simulink library "motohawk_control_primitives_lib"  (Simulink 7.5)
settings: Solver=ode45  SolverMode=SingleTasking  StartTime=0.0  StopTime=10.0  RelTol=1e-3
undefined symbols (not defined in the file): group, motohawk_vardec_config_group, motohawk_vardec_path, p, samp_time, SampleTime
libraries: MotoHawk_lib x103, motohawk_control_primitives_lib x29, simulink x11, AutoDoc_lib x4
(part 4 of 4)

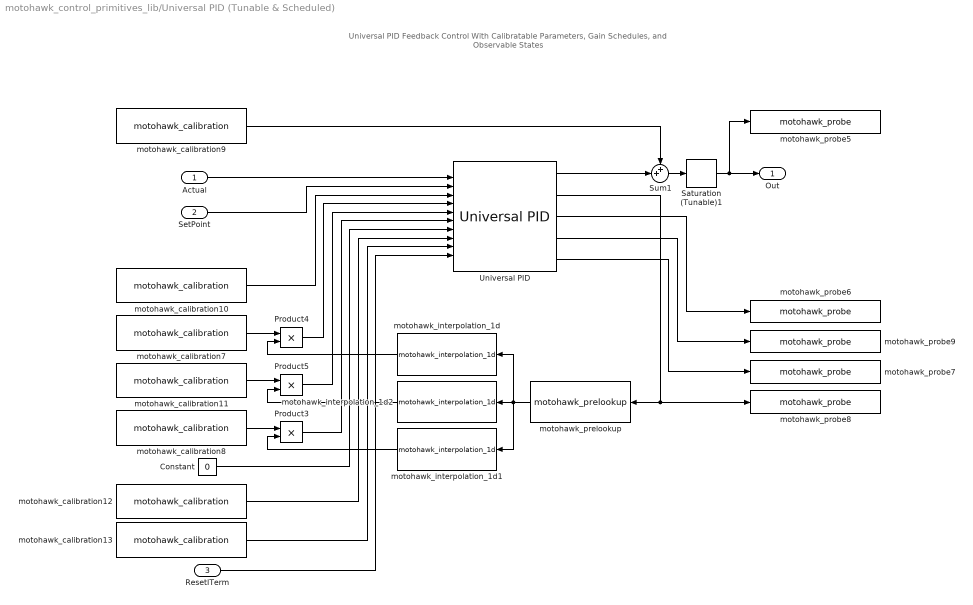
== system motohawk_control_primitives_lib/Universal PID (Tunable & Scheduled) ==
  note: Universal PID Feedback Control
      | With Calibratable Parameters,
      | Gain Schedules, and Observable States
  Actual : Inport  OutDataType=sfix(16)  OutScaling=2^0
  SetPoint : Inport  Port=2  OutDataType=sfix(16)  OutScaling=2^0
  ResetITerm : Inport  Port=3  OutDataType=sfix(16)  OutScaling=2^0
  Constant : Constant  Value=0  OutDataType=sfix(16)  OutScaling=2^0  OutDataTypeStr=Inherit: Inherit via back propagation
  Product3 : Product  OutDataType=sfix(16)  OutScaling=2^0  SaturateOnIntegerOverflow=on  InputSameDT=on  OutDataTypeStr=Inherit: Same as first input
  Product4 : Product  OutDataType=sfix(16)  OutScaling=2^0  SaturateOnIntegerOverflow=on  InputSameDT=on  OutDataTypeStr=Inherit: Same as first input
  Product5 : Product  OutDataType=sfix(16)  OutScaling=2^0  SaturateOnIntegerOverflow=on  InputSameDT=on  OutDataTypeStr=Inherit: Same as first input
  Saturation (Tunable)1 : motohawk_control_primitives_lib/Saturation (Tunable)  prefix=prefix  units=units  grp=motohawk_vardec_config_group(grp)
  Sum1 : Sum  Inputs=++|  OutDataType=sfix(16)  OutScaling=2^0  InputSameDT=on
  Universal PID : motohawk_control_primitives_lib/Universal PID  Description=|  samp_time=SampleTime
      | /* Name: ErrorGain Unit:mult ClassID:VAR StorageID:FLASH Access:RW4+RW3+NA2+NA1 TypeID:UINT4                   
      |    Gain:0.000000001 Min:0.000000000 Max:4.000000000 Format:10.9 UpdateID:REMOTE Help:"This gain is applied to "
      |    "the error term before it is used to calculate the P, I and D terms." VardecSig:6C */                       
      |                                                                                                                
      | /* Name: ITermLowerLim Unit:0 ClassID:VAR StorageID:FLASH Access:RW4+RW3+NA2+NA1 TypeID:SINT2 Gain:0.1         
      |    Min:-3276.8 Max:3276.7 Format:5.1 UpdateID:REMOTE Help:"Lower limit on the I-term value." VardecSig:6C */   
      |                                                                                                                
      | /* Name: ITermUpperLim ClassID:VAR StorageID:FLASH Access:RW4+RW3+NA2+NA1 TypeID:SINT2 Gain:0.1 Min:-3276.8    
      |    Max:3276.7 Format:5.1 UpdateID:REMOTE Help:"Upper limit on I-term value." VardecSig:6C */                   
      |                                                                                                                
      | /* Name: PIDOutLowerLim ClassID:VAR StorageID:FLASH Access:RW4+RW3+NA2+NA1 TypeID:SINT2 Gain:0.1               
      |    Min:-3276.8 Max:3276.7 Format:5.1 UpdateID:REMOTE Help:"Lower limit on PID output." VardecSig:6C */         
      |                                                                                                                
      | /* Name: PIDOutUpperLim ClassID:VAR StorageID:FLASH Access:RW4+RW3+NA2+NA1 TypeID:SINT2 Gain:0.1               
      |    Min:-3276.8 Max:3276.7 Format:3.1 UpdateID:REMOTE Help:"Upper limit on PID output." VardecSig:6C */
  motohawk_calibration10 : MotoHawk_lib/Calibration & Probing Blocks/motohawk_calibration  nam=[prefix 'ErrorGain']  val=1  storage=Calibration  show_more=on  name_source=Use Parameter  data_type=Inherit from 'Default Value'  read_level=1  write_level=1  ovr_cals=on  view_as=Number  enum_struct={'Disabled', 'Enabled'}  vector_style=Wide Row  use_help_units=on  help='PID Error Gain'  units='mult'  use_header_enum=off  row_header_enum={}  col_header_enum={}  use_min_max=off  min_val=-inf  max_val=inf  use_precision=off  precision=''  gain=1  offset=0  exp=1  use_mototune_group=on  mototune_group=motohawk_vardec_config_group(grp)
  motohawk_calibration11 : MotoHawk_lib/Calibration & Probing Blocks/motohawk_calibration  nam=[prefix 'IGain']  val=1  storage=Calibration  show_more=on  name_source=Use Parameter  data_type=Inherit from 'Default Value'  read_level=1  write_level=1  ovr_cals=on  view_as=Number  enum_struct={'Disabled', 'Enabled'}  vector_style=Wide Row  use_help_units=on  help='PID Integrator Gain'  units='mult'  use_header_enum=off  row_header_enum={}  col_header_enum={}  use_min_max=off  min_val=-inf  max_val=inf  use_precision=off  precision=''  gain=1  offset=0  exp=1  use_mototune_group=on  mototune_group=motohawk_vardec_config_group(grp)
  motohawk_calibration12 : MotoHawk_lib/Calibration & Probing Blocks/motohawk_calibration  nam=[prefix 'IMin']  val=0  storage=Calibration  show_more=on  name_source=Use Parameter  data_type=Inherit from 'Default Value'  read_level=1  write_level=1  ovr_cals=on  view_as=Number  enum_struct={'Disabled', 'Enabled'}  vector_style=Wide Row  use_help_units=on  help='PID Integrator Lower Limit'  units=units  use_header_enum=off  row_header_enum={}  col_header_enum={}  use_min_max=off  min_val=-inf  max_val=inf  use_precision=off  precision=''  gain=1  offset=0  exp=1  use_mototune_group=on  mototune_group=motohawk_vardec_config_group(grp)
  motohawk_calibration13 : MotoHawk_lib/Calibration & Probing Blocks/motohawk_calibration  nam=[prefix 'IMax']  val=1  storage=Calibration  show_more=on  name_source=Use Parameter  data_type=Inherit from 'Default Value'  read_level=1  write_level=1  ovr_cals=on  view_as=Number  enum_struct={'Disabled', 'Enabled'}  vector_style=Wide Row  use_help_units=on  help='PID Integrator Upper Limit'  units=units  use_header_enum=off  row_header_enum={}  col_header_enum={}  use_min_max=off  min_val=-inf  max_val=inf  use_precision=off  precision=''  gain=1  offset=0  exp=1  use_mototune_group=on  mototune_group=motohawk_vardec_config_group(grp)
  motohawk_calibration7 : MotoHawk_lib/Calibration & Probing Blocks/motohawk_calibration  nam=[prefix 'PGain']  val=1  storage=Calibration  show_more=on  name_source=Use Parameter  data_type=Inherit from 'Default Value'  read_level=1  write_level=1  ovr_cals=on  view_as=Number  enum_struct={'Disabled', 'Enabled'}  vector_style=Wide Row  use_help_units=on  help='PID Proportional Gain'  units='mult'  use_header_enum=off  row_header_enum={}  col_header_enum={}  use_min_max=off  min_val=-inf  max_val=inf  use_precision=off  precision=''  gain=1  offset=0  exp=1  use_mototune_group=on  mototune_group=motohawk_vardec_config_group(grp)
  motohawk_calibration8 : MotoHawk_lib/Calibration & Probing Blocks/motohawk_calibration  nam=[prefix 'DGain']  val=1  storage=Calibration  show_more=on  name_source=Use Parameter  data_type=Inherit from 'Default Value'  read_level=1  write_level=1  ovr_cals=on  view_as=Number  enum_struct={'Disabled', 'Enabled'}  vector_style=Wide Row  use_help_units=on  help='PID Derivative Gain'  units='mult'  use_header_enum=off  row_header_enum={}  col_header_enum={}  use_min_max=off  min_val=-inf  max_val=inf  use_precision=off  precision=''  gain=1  offset=0  exp=1  use_mototune_group=on  mototune_group=motohawk_vardec_config_group(grp)
  motohawk_calibration9 : MotoHawk_lib/Calibration & Probing Blocks/motohawk_calibration  nam=[prefix 'DCOffset']  val=0  storage=Calibration  show_more=on  name_source=Use Parameter  data_type=Inherit from 'Default Value'  read_level=1  write_level=1  ovr_cals=on  view_as=Number  enum_struct={'Disabled', 'Enabled'}  vector_style=Wide Row  use_help_units=on  help='PID Output DC Offset'  units=units  use_header_enum=off  row_header_enum={}  col_header_enum={}  use_min_max=off  min_val=-inf  max_val=inf  use_precision=off  precision=''  gain=1  offset=0  exp=1  use_mototune_group=on  mototune_group=motohawk_vardec_config_group(grp)
  motohawk_interpolation_1d : MotoHawk_lib/Lookup Tables/motohawk_interpolation_1d  nam=[prefix 'PMult']  table_data=ones(1,tblsize)  show_more=on  data_type=Inherit from 'Table Data'  storage=NonAdaptive  read_level=1  write_level=1  ovr_cals=on  use_help=on  help='Proportional term gain schedule'  units='mult'  use_min_max=off  min_val=-inf  max_val=inf  use_precision=off  precision=''  gain=1  offset=0  exp=1  use_links=off  prelookup_block=''  output_name=''  use_mototune_group=on  mototune_group=grp
  motohawk_interpolation_1d1 : MotoHawk_lib/Lookup Tables/motohawk_interpolation_1d  nam=[prefix 'DMult']  table_data=ones(1,tblsize)  show_more=on  data_type=Inherit from 'Table Data'  storage=NonAdaptive  read_level=1  write_level=1  ovr_cals=on  use_help=on  help='Derivative term gain schedule'  units='mult'  use_min_max=off  min_val=-inf  max_val=inf  use_precision=off  precision=''  gain=1  offset=0  exp=1  use_links=off  prelookup_block=''  output_name=''  use_mototune_group=on  mototune_group=grp
  motohawk_interpolation_1d2 : MotoHawk_lib/Lookup Tables/motohawk_interpolation_1d  nam=[prefix 'IMult']  table_data=ones(1,tblsize)  show_more=on  data_type=Inherit from 'Table Data'  storage=NonAdaptive  read_level=1  write_level=1  ovr_cals=on  use_help=on  help='Integrator term gain schedule'  units='mult'  use_min_max=off  min_val=-inf  max_val=inf  use_precision=off  precision=''  gain=1  offset=0  exp=1  use_links=off  prelookup_block=''  output_name=''  use_mototune_group=on  mototune_group=grp
  motohawk_prelookup : MotoHawk_lib/Lookup Tables/motohawk_prelookup  nam=[prefix 'Error']  breakpoint_data=ones(1,tblsize)  show_more=on  data_type=Inherit from 'Table Data'  storage=Constant  read_level=1  write_level=1  ovr_cals=on  use_help=on  help='Error gain schedule ordinates'  units=units  use_min_max=off  min_val=-inf  max_val=inf  use_precision=off  precision=''  gain=1  offset=0  exp=1  use_links=on  input_name=[prefix 'Error']  use_mototune_group=on  mototune_group=grp
  motohawk_probe5 : MotoHawk_lib/Calibration & Probing Blocks/motohawk_probe  nam=[prefix 'Out']  show_more=on  name_source=Use Parameter  read_level=1  view_as=Number  enum_struct={'Disabled', 'Enabled'}  vector_style=Wide Row  use_help_units=on  help='PID Final Output'  units=units  use_header_enum=off  row_header_enum={}  col_header_enum={}  use_precision=off  precision=''  gain=1  offset=0  exp=1  use_mototune_group=on  mototune_group=grp
  motohawk_probe6 : MotoHawk_lib/Calibration & Probing Blocks/motohawk_probe  nam=[prefix 'PTerm']  show_more=on  name_source=Use Parameter  read_level=1  view_as=Number  enum_struct={'Disabled', 'Enabled'}  vector_style=Wide Row  use_help_units=on  help='PID Proportional Term'  units=units  use_header_enum=off  row_header_enum={}  col_header_enum={}  use_precision=off  precision=''  gain=1  offset=0  exp=1  use_mototune_group=on  mototune_group=grp
  motohawk_probe7 : MotoHawk_lib/Calibration & Probing Blocks/motohawk_probe  nam=[prefix 'DTerm']  show_more=on  name_source=Use Parameter  read_level=1  view_as=Number  enum_struct={'Disabled', 'Enabled'}  vector_style=Wide Row  use_help_units=on  help='PID Derivative Term'  units=units  use_header_enum=off  row_header_enum={}  col_header_enum={}  use_precision=off  precision=''  gain=1  offset=0  exp=1  use_mototune_group=on  mototune_group=grp
  motohawk_probe8 : MotoHawk_lib/Calibration & Probing Blocks/motohawk_probe  nam=[prefix 'Error']  show_more=on  name_source=Use Parameter  read_level=1  view_as=Number  enum_struct={'Disabled', 'Enabled'}  vector_style=Wide Row  use_help_units=on  help='PID Error Term'  units=units  use_header_enum=off  row_header_enum={}  col_header_enum={}  use_precision=off  precision=''  gain=1  offset=0  exp=1  use_mototune_group=on  mototune_group=grp
  motohawk_probe9 : MotoHawk_lib/Calibration & Probing Blocks/motohawk_probe  nam=[prefix 'ITerm']  show_more=on  name_source=Use Parameter  read_level=1  view_as=Number  enum_struct={'Disabled', 'Enabled'}  vector_style=Wide Row  use_help_units=on  help='PID Integrator Term'  units=units  use_header_enum=off  row_header_enum={}  col_header_enum={}  use_precision=off  precision=''  gain=1  offset=0  exp=1  use_mototune_group=on  mototune_group=grp
  Out : Outport  OutDataType=sfix(16)  OutScaling=2^0
  wires:
  motohawk_calibration13/1 -> Universal PID/9
  motohawk_calibration12/1 -> Universal PID/8
  Constant/1 -> Universal PID/7
  ResetITerm/1 -> Universal PID/10
  Universal PID/4 -> motohawk_probe9/1
  Universal PID/3 -> motohawk_probe6/1
  Universal PID/2 -> motohawk_probe8/1, motohawk_prelookup/1
  Product5/1 -> Universal PID/5
  motohawk_interpolation_1d2/1 -> Product5/2
  motohawk_calibration11/1 -> Product5/1
  motohawk_prelookup/1 -> motohawk_interpolation_1d2/1, motohawk_interpolation_1d1/1, motohawk_interpolation_1d/1
  SetPoint/1 -> Universal PID/2
  Actual/1 -> Universal PID/1
  Saturation (Tunable)1/1 -> motohawk_probe5/1, Out/1
  Universal PID/5 -> motohawk_probe7/1
  Universal PID/1 -> Sum1/2
  Sum1/1 -> Saturation (Tunable)1/1
  motohawk_calibration9/1 -> Sum1/1
  motohawk_calibration10/1 -> Universal PID/3
  Product4/1 -> Universal PID/4
  motohawk_calibration7/1 -> Product4/1
  Product3/1 -> Universal PID/6
  motohawk_calibration8/1 -> Product3/1
  motohawk_interpolation_1d/1 -> Product4/2
  motohawk_interpolation_1d1/1 -> Product3/2

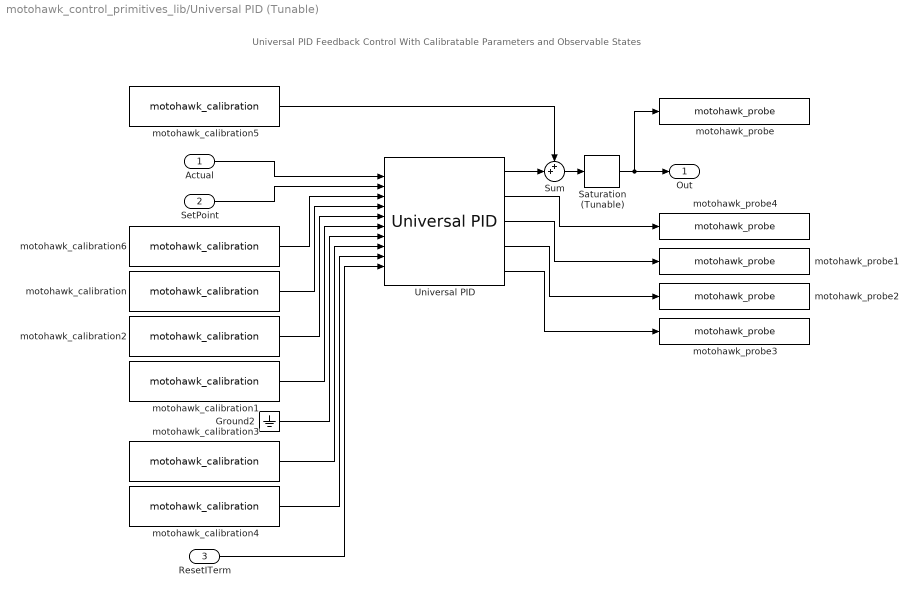
== system motohawk_control_primitives_lib/Universal PID (Tunable) ==
  note: Universal PID Feedback Control
      | With Calibratable Parameters and Observable States
  Actual : Inport  OutDataType=sfix(16)  OutScaling=2^0
  SetPoint : Inport  Port=2  OutDataType=sfix(16)  OutScaling=2^0
  ResetITerm : Inport  Port=3  OutDataType=sfix(16)  OutScaling=2^0
  Ground2 : Ground
  Saturation (Tunable) : motohawk_control_primitives_lib/Saturation (Tunable)  prefix=prefix  units=units  grp=grp
  Sum : Sum  Inputs=++|  OutDataType=sfix(16)  OutScaling=2^0  InputSameDT=on
  Universal PID : motohawk_control_primitives_lib/Universal PID  Description=|  samp_time=SampleTime
      | /* Name: ErrorGain Unit:mult ClassID:VAR StorageID:FLASH Access:RW4+RW3+NA2+NA1 TypeID:UINT4                   
      |    Gain:0.000000001 Min:0.000000000 Max:4.000000000 Format:10.9 UpdateID:REMOTE Help:"This gain is applied to "
      |    "the error term before it is used to calculate the P, I and D terms." VardecSig:6C */                       
      |                                                                                                                
      | /* Name: ITermLowerLim Unit:0 ClassID:VAR StorageID:FLASH Access:RW4+RW3+NA2+NA1 TypeID:SINT2 Gain:0.1         
      |    Min:-3276.8 Max:3276.7 Format:5.1 UpdateID:REMOTE Help:"Lower limit on the I-term value." VardecSig:6C */   
      |                                                                                                                
      | /* Name: ITermUpperLim ClassID:VAR StorageID:FLASH Access:RW4+RW3+NA2+NA1 TypeID:SINT2 Gain:0.1 Min:-3276.8    
      |    Max:3276.7 Format:5.1 UpdateID:REMOTE Help:"Upper limit on I-term value." VardecSig:6C */                   
      |                                                                                                                
      | /* Name: PIDOutLowerLim ClassID:VAR StorageID:FLASH Access:RW4+RW3+NA2+NA1 TypeID:SINT2 Gain:0.1               
      |    Min:-3276.8 Max:3276.7 Format:5.1 UpdateID:REMOTE Help:"Lower limit on PID output." VardecSig:6C */         
      |                                                                                                                
      | /* Name: PIDOutUpperLim ClassID:VAR StorageID:FLASH Access:RW4+RW3+NA2+NA1 TypeID:SINT2 Gain:0.1               
      |    Min:-3276.8 Max:3276.7 Format:3.1 UpdateID:REMOTE Help:"Upper limit on PID output." VardecSig:6C */
  motohawk_calibration : MotoHawk_lib/Calibration & Probing Blocks/motohawk_calibration  nam=[prefix 'PGain']  val=1  storage=Calibration  show_more=on  name_source=Use Parameter  data_type=Inherit from 'Default Value'  read_level=1  write_level=1  ovr_cals=on  view_as=Number  enum_struct={'Disabled', 'Enabled'}  vector_style=Wide Row  use_help_units=on  help='PID Proportional Gain'  units='mult'  use_header_enum=off  row_header_enum={}  col_header_enum={}  use_min_max=off  min_val=-inf  max_val=inf  use_precision=off  precision=''  gain=1  offset=0  exp=1  use_mototune_group=on  mototune_group=grp
  motohawk_calibration1 : MotoHawk_lib/Calibration & Probing Blocks/motohawk_calibration  nam=[prefix 'DGain']  val=1  storage=Calibration  show_more=on  name_source=Use Parameter  data_type=Inherit from 'Default Value'  read_level=1  write_level=1  ovr_cals=on  view_as=Number  enum_struct={'Disabled', 'Enabled'}  vector_style=Wide Row  use_help_units=on  help='PID Derivative Gain'  units='mult'  use_header_enum=off  row_header_enum={}  col_header_enum={}  use_min_max=off  min_val=-inf  max_val=inf  use_precision=off  precision=''  gain=1  offset=0  exp=1  use_mototune_group=on  mototune_group=grp
  motohawk_calibration2 : MotoHawk_lib/Calibration & Probing Blocks/motohawk_calibration  nam=[prefix 'IGain']  val=1  storage=Calibration  show_more=on  name_source=Use Parameter  data_type=Inherit from 'Default Value'  read_level=1  write_level=1  ovr_cals=on  view_as=Number  enum_struct={'Disabled', 'Enabled'}  vector_style=Wide Row  use_help_units=on  help='PID Integral Gain'  units='mult'  use_header_enum=off  row_header_enum={}  col_header_enum={}  use_min_max=off  min_val=-inf  max_val=inf  use_precision=off  precision=''  gain=1  offset=0  exp=1  use_mototune_group=on  mototune_group=grp
  motohawk_calibration3 : MotoHawk_lib/Calibration & Probing Blocks/motohawk_calibration  nam=[prefix 'IMin']  val=0  storage=Calibration  show_more=on  name_source=Use Parameter  data_type=Inherit from 'Default Value'  read_level=1  write_level=1  ovr_cals=on  view_as=Number  enum_struct={'Disabled', 'Enabled'}  vector_style=Wide Row  use_help_units=on  help='PID Integrator Lower Limit'  units=units  use_header_enum=off  row_header_enum={}  col_header_enum={}  use_min_max=off  min_val=-inf  max_val=inf  use_precision=off  precision=''  gain=1  offset=0  exp=1  use_mototune_group=on  mototune_group=grp
  motohawk_calibration4 : MotoHawk_lib/Calibration & Probing Blocks/motohawk_calibration  nam=[prefix 'IMax']  val=1  storage=Calibration  show_more=on  name_source=Use Parameter  data_type=Inherit from 'Default Value'  read_level=1  write_level=1  ovr_cals=on  view_as=Number  enum_struct={'Disabled', 'Enabled'}  vector_style=Wide Row  use_help_units=on  help='PID Integrator Upper Limit'  units=units  use_header_enum=off  row_header_enum={}  col_header_enum={}  use_min_max=off  min_val=-inf  max_val=inf  use_precision=off  precision=''  gain=1  offset=0  exp=1  use_mototune_group=on  mototune_group=grp
  motohawk_calibration5 : MotoHawk_lib/Calibration & Probing Blocks/motohawk_calibration  nam=[prefix 'DCOffset']  val=0  storage=Calibration  show_more=on  name_source=Use Parameter  data_type=Inherit from 'Default Value'  read_level=1  write_level=1  ovr_cals=on  view_as=Number  enum_struct={'Disabled', 'Enabled'}  vector_style=Wide Row  use_help_units=on  help='PID Output DC Offset'  units=units  use_header_enum=off  row_header_enum={}  col_header_enum={}  use_min_max=off  min_val=-inf  max_val=inf  use_precision=off  precision=''  gain=1  offset=0  exp=1  use_mototune_group=on  mototune_group=grp
  motohawk_calibration6 : MotoHawk_lib/Calibration & Probing Blocks/motohawk_calibration  nam=[prefix 'ErrorGain']  val=1  storage=Calibration  show_more=on  name_source=Use Parameter  data_type=Inherit from 'Default Value'  read_level=1  write_level=1  ovr_cals=on  view_as=Number  enum_struct={'Disabled', 'Enabled'}  vector_style=Wide Row  use_help_units=on  help='PID Error Gain'  units='mult'  use_header_enum=off  row_header_enum={}  col_header_enum={}  use_min_max=off  min_val=-inf  max_val=inf  use_precision=off  precision=''  gain=1  offset=0  exp=1  use_mototune_group=on  mototune_group=grp
  motohawk_probe : MotoHawk_lib/Calibration & Probing Blocks/motohawk_probe  nam=[prefix 'Out']  show_more=on  name_source=Use Parameter  read_level=1  view_as=Number  enum_struct={'Disabled', 'Enabled'}  vector_style=Wide Row  use_help_units=on  help='PID Final Output'  units=units  use_header_enum=off  row_header_enum={}  col_header_enum={}  use_precision=off  precision=''  gain=1  offset=0  exp=1  use_mototune_group=on  mototune_group=grp
  motohawk_probe1 : MotoHawk_lib/Calibration & Probing Blocks/motohawk_probe  nam=[prefix 'PTerm']  show_more=on  name_source=Use Parameter  read_level=1  view_as=Number  enum_struct={'Disabled', 'Enabled'}  vector_style=Wide Row  use_help_units=on  help='PID Proportional Term'  units=units  use_header_enum=off  row_header_enum={}  col_header_enum={}  use_precision=off  precision=''  gain=1  offset=0  exp=1  use_mototune_group=on  mototune_group=grp
  motohawk_probe2 : MotoHawk_lib/Calibration & Probing Blocks/motohawk_probe  nam=[prefix 'ITerm']  show_more=on  name_source=Use Parameter  read_level=1  view_as=Number  enum_struct={'Disabled', 'Enabled'}  vector_style=Wide Row  use_help_units=on  help='PID Integrator Term'  units=units  use_header_enum=off  row_header_enum={}  col_header_enum={}  use_precision=off  precision=''  gain=1  offset=0  exp=1  use_mototune_group=on  mototune_group=grp
  motohawk_probe3 : MotoHawk_lib/Calibration & Probing Blocks/motohawk_probe  nam=[prefix 'DTerm']  show_more=on  name_source=Use Parameter  read_level=1  view_as=Number  enum_struct={'Disabled', 'Enabled'}  vector_style=Wide Row  use_help_units=on  help='PID Derivative Term'  units=units  use_header_enum=off  row_header_enum={}  col_header_enum={}  use_precision=off  precision=''  gain=1  offset=0  exp=1  use_mototune_group=on  mototune_group=grp
  motohawk_probe4 : MotoHawk_lib/Calibration & Probing Blocks/motohawk_probe  nam=[prefix 'Error']  show_more=on  name_source=Use Parameter  read_level=1  view_as=Number  enum_struct={'Disabled', 'Enabled'}  vector_style=Wide Row  use_help_units=on  help='PID Error Term'  units=units  use_header_enum=off  row_header_enum={}  col_header_enum={}  use_precision=off  precision=''  gain=1  offset=0  exp=1  use_mototune_group=on  mototune_group=grp
  Out : Outport  OutDataType=sfix(16)  OutScaling=2^0
  wires:
  motohawk_calibration5/1 -> Sum/1
  Sum/1 -> Saturation (Tunable)/1
  ResetITerm/1 -> Universal PID/10
  Ground2/1 -> Universal PID/7
  motohawk_calibration1/1 -> Universal PID/6
  motohawk_calibration2/1 -> Universal PID/5
  motohawk_calibration/1 -> Universal PID/4
  Universal PID/3 -> motohawk_probe1/1
  Actual/1 -> Universal PID/1
  SetPoint/1 -> Universal PID/2
  Universal PID/1 -> Sum/2
  motohawk_calibration6/1 -> Universal PID/3
  motohawk_calibration3/1 -> Universal PID/8
  motohawk_calibration4/1 -> Universal PID/9
  Universal PID/4 -> motohawk_probe2/1
  Universal PID/5 -> motohawk_probe3/1
  Universal PID/2 -> motohawk_probe4/1
  Saturation (Tunable)/1 -> Out/1, motohawk_probe/1

== system motohawk_control_primitives_lib/Variable Rate Limiter ==
  note: Rate Limiter - Limit allowable change in signal per timestep
  input : Inport  OutDataType=sfix(16)  OutScaling=2^0
  rise rate : Inport  Port=2  OutDataType=sfix(16)  OutScaling=2^0
  fall rate : Inport  Port=3  OutDataType=sfix(16)  OutScaling=2^0
  Product : Product  OutDataType=sfix(16)  OutScaling=2^0  SaturateOnIntegerOverflow=on  InputSameDT=on  OutDataTypeStr=Inherit: Same as first input
  Product1 : Product  Inputs=/*  OutDataType=sfix(16)  OutScaling=2^0  SaturateOnIntegerOverflow=on  InputSameDT=on  OutDataTypeStr=Inherit: Same as first input
  Saturation : motohawk_control_primitives_lib/Saturation
  Sum2 : Sum  Inputs=|++  OutDataType=sfix(16)  OutScaling=2^0  SaturateOnIntegerOverflow=on  InputSameDT=on  OutDataTypeStr=Inherit: Same as first input
  Sum3 : Sum  Inputs=|+-  OutDataType=sfix(16)  OutScaling=2^0  SaturateOnIntegerOverflow=on  InputSameDT=on  OutDataTypeStr=Inherit: Same as first input
  Unit Delay : UnitDelay  SampleTime=-1
  motohawk_delta_time : MotoHawk_lib/Extra Development Blocks/motohawk_delta_time  samp_time=-1  init_val=.005
  output : Outport  OutDataType=sfix(16)  OutScaling=2^0  InitialOutput=0
  wires:
  Saturation/1 -> Product/2
  input/1 -> Sum3/1
  Product1/1 -> Saturation/1  "Slope"
  Unit Delay/1 -> Sum3/2, Sum2/2
  Sum2/1 -> Unit Delay/1, output/1
  Product/1 -> Sum2/1
  fall rate/1 -> Saturation/2  "Lo Lim"
  rise rate/1 -> Saturation/3  "Hi Lim"
  Sum3/1 -> Product1/2
  motohawk_delta_time/1 -> Product1/1, Product/1

== system motohawk_control_primitives_lib/Hysterisis/Hysteresis ==
  note: Hi & !Lo => Hi
      | Lo & !Hi => Lo
      | Otherwise, Hold
  Hi : Inport  OutDataType=sfix(16)  OutScaling=2^0
  Lo : Inport  Port=2  OutDataType=sfix(16)  OutScaling=2^0
  Combinatorial  Logic : CombinatorialLogic  TruthTable=[0 0;0 1;1 1;0 0]
  Demux : Demux  Outputs=2
  Mux : Mux  Inputs=2
  Switch1 : Switch  Threshold=0.5  SaturateOnIntegerOverflow=on  InputSameDT=on
  Unit Delay : UnitDelay  SampleTime=-1
  "Out (Lo=0, Hi=1)" : Outport  OutDataType=sfix(16)  OutScaling=2^0
  wires:
  Mux/1 -> Combinatorial  Logic/1
  Combinatorial  Logic/1 -> Demux/1
  Demux/1 -> Switch1/1
  Demux/2 -> Switch1/2
  Unit Delay/1 -> Switch1/3
  Switch1/1 -> Unit Delay/1, "Out (Lo=0, Hi=1)"/1
  Hi/1 -> Mux/1
  Lo/1 -> Mux/2

== system motohawk_control_primitives_lib/Inc_DecFilterSelect1/DecreasingFilter ==
  Enable : EnablePort
  motohawk_calibration2 : MotoHawk_lib/Calibration & Probing Blocks/motohawk_calibration  nam=[nam 'DecFiltC']  val=1.25  storage=Calibration  show_more=on  name_source=Use Parameter  data_type=Inherit from 'Default Value'  read_level=1  write_level=1  ovr_cals=on  view_as=Number  enum_struct={'Disabled', 'Enabled'}  vector_style=Wide Row  use_help_units=on  help='Filter time constant for a decreasing signal.'  units='sec'  use_header_enum=off  row_header_enum={}  col_header_enum={}  use_min_max=off  min_val=-inf  max_val=inf  use_precision=off  precision=''  gain=1  offset=0  exp=1  use_mototune_group=on  mototune_group=grp_cal
  Out1 : Outport  OutDataType=sfix(16)  OutScaling=2^0  InitialOutput=.005
  wires:
  motohawk_calibration2/1 -> Out1/1

== system motohawk_control_primitives_lib/Inc_DecFilterSelect1/IncreasingFilter ==
  Enable : EnablePort
  motohawk_calibration1 : MotoHawk_lib/Calibration & Probing Blocks/motohawk_calibration  nam=[nam 'IncFiltC']  val=1.25  storage=Calibration  show_more=on  name_source=Use Parameter  data_type=Inherit from 'Default Value'  read_level=1  write_level=1  ovr_cals=on  view_as=Number  enum_struct={'Disabled', 'Enabled'}  vector_style=Wide Row  use_help_units=on  help='Filter time constant for a increasing signal.'  units='sec'  use_header_enum=off  row_header_enum={}  col_header_enum={}  use_min_max=off  min_val=-inf  max_val=inf  use_precision=off  precision=''  gain=1  offset=0  exp=1  use_mototune_group=on  mototune_group=grp_cal
  Out1 : Outport  OutDataType=sfix(16)  OutScaling=2^0  InitialOutput=.005
  wires:
  motohawk_calibration1/1 -> Out1/1

== system motohawk_control_primitives_lib/Per Cylinder Tables/Cyl1 ==
  Row : Inport  OutDataType=sfix(16)  OutScaling=2^0
  Col : Inport  Port=2  OutDataType=sfix(16)  OutScaling=2^0
  Action Port : ActionPort
  motohawk_interpolation_2d : MotoHawk_lib/Lookup Tables/motohawk_interpolation_2d  nam=[nam 'Cyl1']  table_data=table1data  show_more=on  read_level=1  write_level=1  use_help=off  help=''  units=''  use_precision=off  precision=''  gain=1  offset=0  exp=1  use_links=on  row_prelookup_block=rowprelookup  col_prelookup_block=colprelookup  output_name=''  use_mototune_group=on  mototune_group=grp
  Value : Outport  OutDataType=sfix(16)  OutScaling=2^0
  wires:
  motohawk_interpolation_2d/1 -> Value/1
  Col/1 -> motohawk_interpolation_2d/2
  Row/1 -> motohawk_interpolation_2d/1

== system motohawk_control_primitives_lib/Per Cylinder Tables/Cyl2 ==
  Row : Inport  OutDataType=sfix(16)  OutScaling=2^0
  Col : Inport  Port=2  OutDataType=sfix(16)  OutScaling=2^0
  Action Port : ActionPort
  motohawk_interpolation_2d1 : MotoHawk_lib/Lookup Tables/motohawk_interpolation_2d  nam=[nam 'Cyl2']  table_data=table2data  show_more=on  read_level=1  write_level=1  use_help=off  help=''  units=''  use_precision=off  precision=''  gain=1  offset=0  exp=1  use_links=on  row_prelookup_block=rowprelookup  col_prelookup_block=colprelookup  output_name=''  use_mototune_group=on  mototune_group=grp
  Value : Outport  OutDataType=sfix(16)  OutScaling=2^0
  wires:
  motohawk_interpolation_2d1/1 -> Value/1
  Col/1 -> motohawk_interpolation_2d1/2
  Row/1 -> motohawk_interpolation_2d1/1

== system motohawk_control_primitives_lib/Per Cylinder Tables/Cyl3 ==
  Row : Inport  OutDataType=sfix(16)  OutScaling=2^0
  Col : Inport  Port=2  OutDataType=sfix(16)  OutScaling=2^0
  Action Port : ActionPort
  motohawk_interpolation_2d2 : MotoHawk_lib/Lookup Tables/motohawk_interpolation_2d  nam=[nam 'Cyl3']  table_data=table3data  show_more=on  read_level=1  write_level=1  use_help=off  help=''  units=''  use_precision=off  precision=''  gain=1  offset=0  exp=1  use_links=on  row_prelookup_block=rowprelookup  col_prelookup_block=colprelookup  output_name=''  use_mototune_group=on  mototune_group=grp
  Value : Outport  OutDataType=sfix(16)  OutScaling=2^0
  wires:
  motohawk_interpolation_2d2/1 -> Value/1
  Col/1 -> motohawk_interpolation_2d2/2
  Row/1 -> motohawk_interpolation_2d2/1

== system motohawk_control_primitives_lib/Per Cylinder Tables/Cyl4 ==
  Row : Inport  OutDataType=sfix(16)  OutScaling=2^0
  Col : Inport  Port=2  OutDataType=sfix(16)  OutScaling=2^0
  Action Port : ActionPort
  motohawk_interpolation_2d3 : MotoHawk_lib/Lookup Tables/motohawk_interpolation_2d  nam=[nam 'Cyl4']  table_data=table4data  show_more=on  read_level=1  write_level=1  use_help=off  help=''  units=''  use_precision=off  precision=''  gain=1  offset=0  exp=1  use_links=on  row_prelookup_block=rowprelookup  col_prelookup_block=colprelookup  output_name=''  use_mototune_group=on  mototune_group=grp
  Value : Outport  OutDataType=sfix(16)  OutScaling=2^0
  wires:
  motohawk_interpolation_2d3/1 -> Value/1
  Col/1 -> motohawk_interpolation_2d3/2
  Row/1 -> motohawk_interpolation_2d3/1

== system motohawk_control_primitives_lib/Per Cylinder Tables/Cyl5 ==
  Row : Inport  OutDataType=sfix(16)  OutScaling=2^0
  Col : Inport  Port=2  OutDataType=sfix(16)  OutScaling=2^0
  Action Port : ActionPort
  motohawk_interpolation_2d4 : MotoHawk_lib/Lookup Tables/motohawk_interpolation_2d  nam=[nam 'Cyl5']  table_data=table5data  show_more=on  read_level=1  write_level=1  use_help=off  help=''  units=''  use_precision=off  precision=''  gain=1  offset=0  exp=1  use_links=on  row_prelookup_block=rowprelookup  col_prelookup_block=colprelookup  output_name=''  use_mototune_group=on  mototune_group=grp
  Value : Outport  OutDataType=sfix(16)  OutScaling=2^0
  wires:
  motohawk_interpolation_2d4/1 -> Value/1
  Col/1 -> motohawk_interpolation_2d4/2
  Row/1 -> motohawk_interpolation_2d4/1

== system motohawk_control_primitives_lib/Per Cylinder Tables/Cyl6 ==
  Row : Inport  OutDataType=sfix(16)  OutScaling=2^0
  Col : Inport  Port=2  OutDataType=sfix(16)  OutScaling=2^0
  Action Port : ActionPort
  motohawk_interpolation_2d5 : MotoHawk_lib/Lookup Tables/motohawk_interpolation_2d  nam=[nam 'Cyl6']  table_data=(table6data)  show_more=on  read_level=1  write_level=1  use_help=off  help=''  units=''  use_precision=off  precision=''  gain=1  offset=0  exp=1  use_links=on  row_prelookup_block=rowprelookup  col_prelookup_block=colprelookup  output_name=''  use_mototune_group=on  mototune_group=grp
  Value : Outport  OutDataType=sfix(16)  OutScaling=2^0
  wires:
  motohawk_interpolation_2d5/1 -> Value/1
  Col/1 -> motohawk_interpolation_2d5/2
  Row/1 -> motohawk_interpolation_2d5/1

== system motohawk_control_primitives_lib/Polynomial (Tunable)/Horner's Rule ==
  note: Horner's Rule.
  u_hat : Inport  OutDataType=sfix(16)  OutScaling=2^0
  p : Inport  Port=2  OutDataType=sfix(16)  OutScaling=2^0
  Constant : Constant  OutDataType=sfix(16)  OutScaling=2^0  OutDataTypeStr=Inherit: Inherit via back propagation
  Direct Look-Up Table (n-D) : simulink/Lookup Tables/Direct Lookup Table (n-D)  maskTabDims=1  explicitNumDims=1  outDims=Element  tabIsInput=on  mxTable=[4 5 6;16 19 20;10 18 23]  clipFlag=None
  For Iterator : ForIterator  ResetStates=reset  IterationLimit=length(p)
  Product1 : Product  OutDataType=sfix(16)  OutScaling=2^0  SaturateOnIntegerOverflow=on  OutDataTypeStr=Inherit: Same as first input
  Sum0 : Sum  Inputs=|+-  OutDataType=sfix(16)  OutScaling=2^0  OutDataTypeStr=Inherit: Inherit via back propagation  SaturateOnIntegerOverflow=on  InputSameDT=on
  Sum1 : Sum  Inputs=|++  OutDataType=sfix(16)  OutScaling=2^0  OutDataTypeStr=Inherit: Inherit via back propagation  SaturateOnIntegerOverflow=on  InputSameDT=on
  Unit Delay : UnitDelay  SampleTime=-1
  y : Outport  OutDataType=sfix(16)  OutScaling=2^0
  wires:
  p/1 -> Direct Look-Up Table (n-D)/2
  u_hat/1 -> Product1/2
  Constant/1 -> Sum0/2
  Sum0/1 -> Direct Look-Up Table (n-D)/1
  Unit Delay/1 -> Product1/1
  Product1/1 -> Sum1/1
  Direct Look-Up Table (n-D)/1 -> Sum1/2
  Sum1/1 -> Unit Delay/1, y/1
  For Iterator/1 -> Sum0/1

== system motohawk_control_primitives_lib/Saturate Divide/Normal Divide ==
  X : Inport  OutDataType=sfix(16)  OutScaling=2^0
  Inport : Inport  Port=2  OutDataType=sfix(16)  OutScaling=2^0
  Divisor OK : ActionPort  InitializeStates=reset  ActionType=else
  Product : Product  Inputs=*/  OutDataType=sfix(16)  OutScaling=2^0  SaturateOnIntegerOverflow=on  InputSameDT=on  OutDataTypeStr=Inherit: Same as first input
  " " : Outport  OutDataType=sfix(16)  OutScaling=2^0
  wires:
  X/1 -> Product/1
  Product/1 -> " "/1
  ? -> Product/2

== system motohawk_control_primitives_lib/Saturate Divide/Output One ==
  Action Port : ActionPort  ActionType=then
  Constant : Constant  OutDataType=sfix(16)  OutScaling=2^0  OutDataTypeStr=Inherit: Inherit via back propagation
  " " : Outport  OutDataType=sfix(16)  OutScaling=2^0
  wires:
  Constant/1 -> " "/1
